simulink model "MX28kinematics"  (R2014b)
settings: Solver=ode15s  StartTime=0.0  StopTime=0.5  RelTol=1e-3
undefined symbols (not defined in the file or in its folder): MX28_inertia, MX28_Te
libraries: sm_lib x5, nesl_utility x4, fl_lib x2
settings Model: Creator=florent  LastModifiedBy=florent
settings DebuggingCC: IntegerOverflowMsg=none  ParameterDowncastMsg=warning  ParameterPrecisionLossMsg=none  ParameterTunabilityLossMsg=none  StateNameClashWarn=warning  IntegerSaturationMsg=none

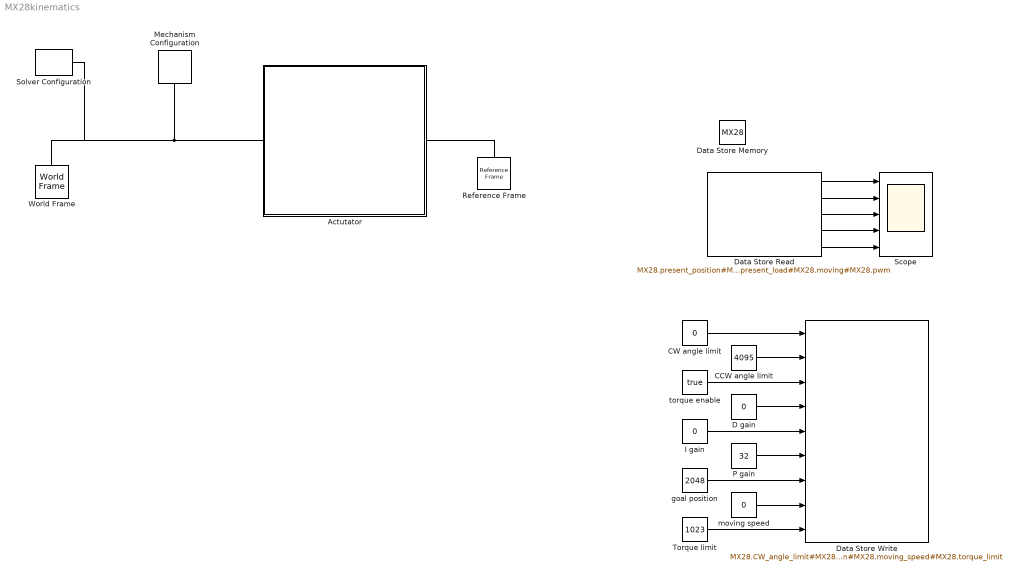
== system MX28kinematics ==
  Actutator : Subsystem
  CCW angle limit : Constant  Value=4095  OutDataTypeStr=int16
  CW angle limit : Constant  Value=0  OutDataTypeStr=int16
  D gain : Constant  Value=0  OutDataTypeStr=uint8
  Data Store Memory : DataStoreMemory  DataStoreName=MX28  WriteAfterWriteMsg=error  InitialValue=MX28_default  VectorParams1D=off  OutDataTypeStr=Bus: MX28_bus
  Data Store Read : DataStoreRead  DataStoreName=MX28  SampleTime=0.001  DataStoreElements=MX28.present_position#MX28.present_speed#MX28.present_load#MX28.moving#MX28.pwm
  Data Store Write : DataStoreWrite  DataStoreName=MX28  DataStoreElements=MX28.CW_angle_limit#MX28.CCW_angle_limit#MX28.torque_enable#MX28.D_gain#MX28.I_gain#MX28.P_gain#MX28.goal_position#MX28.moving_speed#MX28.torque_limit
  I gain : Constant  Value=0  OutDataTypeStr=uint8
  Mechanism Configuration : sm_lib/Utilities/Mechanism Configuration  UniformGravity=Constant  GravityVector=[0 0 -9.80665]  GravityUnits=m/s^2  LinearizationDelta=0.001  BlockFunction=simmechanics.library.utilities.mechanism_configuration
  P gain : Constant  Value=32  OutDataTypeStr=uint8
  Reference Frame : sm_lib/Frames and Transforms/Reference Frame  BlockFunction=simmechanics.library.frames_transforms.reference_frame
  Scope : Scope  NumInputPorts=5
      settings: YMin=1900~-600~-1000~0~-5  YMax=2050~0~500~1~5
  Solver Configuration : nesl_utility/Solver Configuration  PhysicalDomain=network_engine_domain  SubClassName=solver  LeftPortType=input  RightPortType=generic  Accelerate=off  Tones=[]  Harmonics=[]  SimulateNoise=off  Profile=off  UseLocalSampling=off  EnableSwitchedLinearOptims=on  FrequencyDomain=off  UseCCode=off  RelTol=0.001  AbsTol=1e-06  MinStep=1e-09  ToWorkspace=off  DoDC=off  ResidualTolerance=1e-09  UseLocalSolver=off  LocalSolverChoice=NE_BACKWARD_EULER_ADVANCER  LocalSolverSampleTime=0.001  DoFixedCost=off  MaxNonlinIter=3  MaxModeIter=2  LinearAlgebra=Sparse  DelaysMemoryBudget=1024  AutomaticFiltering=on  FilteringTimeConstant=0.001
  Torque limit : Constant  Value=1023  OutDataTypeStr=int16
  World Frame : sm_lib/Frames and Transforms/World Frame  BlockFunction=simmechanics.library.frames_transforms.world_frame
  goal position : Constant  Value=2048  OutDataTypeStr=int16
  moving speed : Constant  Value=0  OutDataTypeStr=int16
  torque enable : Constant  Value=true  OutDataTypeStr=boolean
  wires:
  Data Store Read/1 -> Scope/1
  Data Store Read/2 -> Scope/2
  Data Store Read/3 -> Scope/3
  Data Store Read/4 -> Scope/4
  Data Store Read/5 -> Scope/5
  Torque limit/1 -> Data Store Write/9
  moving speed/1 -> Data Store Write/8
  goal position/1 -> Data Store Write/7
  P gain/1 -> Data Store Write/6
  I gain/1 -> Data Store Write/5
  D gain/1 -> Data Store Write/4
  torque enable/1 -> Data Store Write/3
  CW angle limit/1 -> Data Store Write/1
  CCW angle limit/1 -> Data Store Write/2
  connections:
  Reference Frame/RConn1 -- Actutator/RConn1
  Mechanism Configuration/RConn1 -- Actutator/LConn1 -- Solver Configuration/RConn1 -- World Frame/RConn1

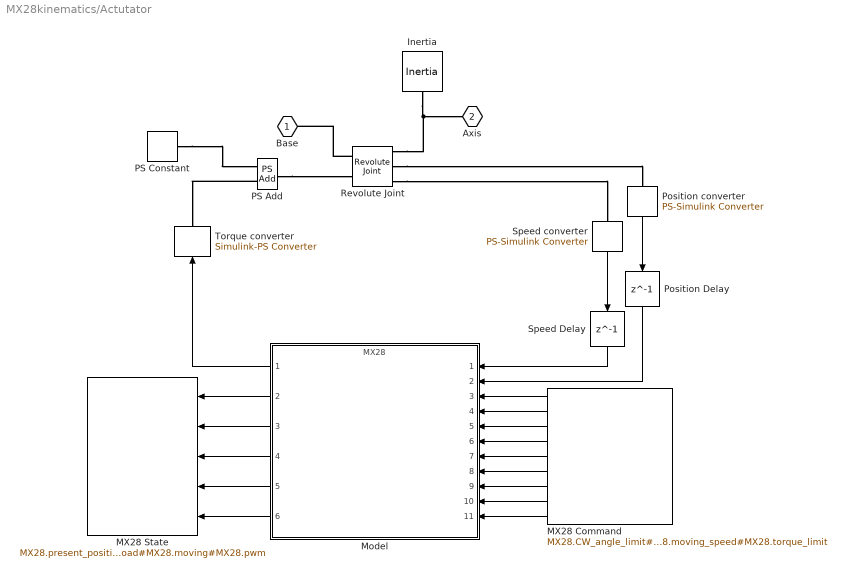
== system MX28kinematics/Actutator ==
  Inertia : sm_lib/Body Elements/Inertia  InertiaType=Custom  Mass=1  MassUnits=g  CenterOfMass=[0 0 0]  CenterOfMassUnits=m  MomentsOfInertia=[0 0 MX28_inertia]  MomentsOfInertiaUnits=kg*m^2  ProductsOfInertia=[0 0 0]  ProductsOfInertiaUnits=kg*m^2  BlockFunction=simmechanics.library.body_elements.inertia
  MX28 Command : DataStoreRead  DataStoreName=MX28  SampleTime=MX28_Te  DataStoreElements=MX28.CW_angle_limit#MX28.CCW_angle_limit#MX28.torque_enable#MX28.D_gain#MX28.I_gain#MX28.P_gain#MX28.goal_position#MX28.moving_speed#MX28.torque_limit
  MX28 State : DataStoreWrite  DataStoreName=MX28  DataStoreElements=MX28.present_position#MX28.present_speed#MX28.present_load#MX28.moving#MX28.pwm
  Model : ModelReference  ModelNameDialog=MX28.slx  SimulationMode=Normal  ModelReferenceVersion=1.66  CopyOfModelName=MX28.slx  DefaultDataLogging=on
  PS Add : fl_lib/Physical Signals/Functions/PS Add
  PS Constant : fl_lib/Physical Signals/Sources/PS Constant  constant=0
  Position Delay : Delay  DelayLength=1  InitialCondition=pi  SampleTime=MX28_Te
  Position converter : nesl_utility/PS-Simulink Converter  PhysicalDomain=network_engine_domain  SubClassName=ps_output  LeftPortType=input  RightPortType=output  PseudoPeriodic=off  Frequencies=[]  Unit=rad  AffineConversion=off
  Revolute Joint : sm_lib/Joints/Revolute Joint  SenseConstraintForce=off  SenseConstraintForceX=off  SenseConstraintForceY=off  SenseConstraintForceZ=off  SenseConstraintTorque=off  SenseConstraintTorqueX=off  SenseConstraintTorqueY=off  SenseConstraintTorqueZ=off  SenseTotalForce=off  SenseTotalForceX=off  SenseTotalForceY=off  SenseTotalForceZ=off  SenseTotalTorque=off  SenseTotalTorqueX=off  SenseTotalTorqueY=off  SenseTotalTorqueZ=off  CompositeWrenchDir=FollowerOnBase  CompositeWrenchFrame=BaseFrame  EquilibriumPosition=0  EquilibriumPositionUnits=deg  SpringStiffness=0  SpringStiffnessUnits=N*m/deg  DampingCoefficient=MX28_lub_friction  DampingCoefficientUnits=N*m/(rad/s)  TorqueActuationMode=InputTorque  MotionActuationMode=ComputedMotion  SensePosition=on  SenseVelocity=on  SenseAcceleration=off  SenseTorqueForce=off  PositionTargetValue=180  PositionTargetValueUnits=deg  PositionTargetSpecify=on  PositionTargetPriority=High  VelocityTargetValue=0  VelocityTargetValueUnits=deg/s  VelocityTargetSpecify=off  VelocityTargetPriority=High  BlockFunction=simmechanics.library.joints.revolute_joint
  Speed Delay : Delay  DelayLength=1  SampleTime=MX28_Te
  Speed converter : nesl_utility/PS-Simulink Converter  PhysicalDomain=network_engine_domain  SubClassName=ps_output  LeftPortType=input  RightPortType=output  PseudoPeriodic=off  Frequencies=[]  Unit=rad/s  AffineConversion=off
  Torque converter : nesl_utility/Simulink-PS Converter  PhysicalDomain=network_engine_domain  SubClassName=ps_input  LeftPortType=input  RightPortType=output  PseudoPeriodic=off  Frequencies=[]  NoiseDistribution=none  NoiseParameters=[]  Unit=N*m  AffineConversion=off  InputFiltering=off  SimscapeFilterOrder=1  InputFilterTimeConstant=0.001  UdotUserProvided=1
  Base : PMIOPort  Port=1  Side=Left
  Axis : PMIOPort  Port=2  Side=Right
  wires:
  Model/4 -> MX28 State/3
  Model/2 -> MX28 State/1
  Model/5 -> MX28 State/4
  Model/3 -> MX28 State/2
  Model/1 -> Torque converter/1
  Speed converter/1 -> Speed Delay/1
  Position converter/1 -> Position Delay/1
  MX28 Command/3 -> Model/5
  MX28 Command/6 -> Model/8
  MX28 Command/4 -> Model/6
  MX28 Command/5 -> Model/7
  MX28 Command/7 -> Model/9
  MX28 Command/2 -> Model/4
  MX28 Command/1 -> Model/3
  Speed Delay/1 -> Model/1
  Position Delay/1 -> Model/2
  Model/6 -> MX28 State/5
  MX28 Command/8 -> Model/10
  MX28 Command/9 -> Model/11
  connections:
  Revolute Joint/LConn1 -- Base/RConn1
  Revolute Joint/RConn1 -- Axis/RConn1 -- Inertia/RConn1
  Revolute Joint/RConn2 -- Position converter/LConn1
  Revolute Joint/RConn3 -- Speed converter/LConn1
  PS Add/RConn1 -- Revolute Joint/LConn2
  PS Add/LConn2 -- Torque converter/RConn1
  PS Constant/RConn1 -- PS Add/LConn1
